simulink library "lib_transmission2"  (Simulink 4.1.1)
values from neighbouring files (symbols this model uses):
  logFlag = 1    [advSACompMaskInit.m]    (also in advSACompMaskInitR13.m)
undefined symbols (not defined in the file or in its folder): cyc_mph, fc_map_spd, fc_max_trq, fc_spd_scale, fc_trq_scale, fd_inertia, fd_loss, fd_ratio, gb_dnshift_load, gb_dnshift_spd, gb_gear_number_lookup, gb_gears_num, gb_inertia, gb_loss_const, gb_loss_input_spd_coeff, gb_loss_input_trq_coeff, gb_loss_output_spd_coeff, gb_loss_output_trq_coeff, gb_map_spd_out, gb_map_trq_in, gb_map_trq_out, gb_num_init, gb_ratio, gb_shift_delay, gb_spd_scale, gb_trq_scale, gb_upshift_load, gb_upshift_spd, htc_inertia, htc_k_adv, htc_k_adv_coast, htc_lockup, htc_lockup_load, htc_lockup_spd, htc_lu_gear_range, htc_max_coast_tr, htc_min_coast_tr, htc_pump_loss_spd, htc_pump_loss_trq_lockup, htc_pump_loss_trq_unlock, htc_sr, htc_sr_coast, htc_tr, htc_tr_coast, htc_unlock_spd, mc_map_spd, mc_max_trq, mc_overtrq_factor, mc_spd_scale, mc_trq_scale, tc_loss, tc_mc_to_fc_ratio, tx_eff_map, tx_map_spd, tx_map_trq, tx_pg_r, tx_pg_s, tx_speed_dep, vc_clutch_bool, vc_idle_spd ... (+2)
libraries: lib_controls x1, lib_etc x1, lib_controls2 x1, lib_transmission x1
(part 7 of 17)

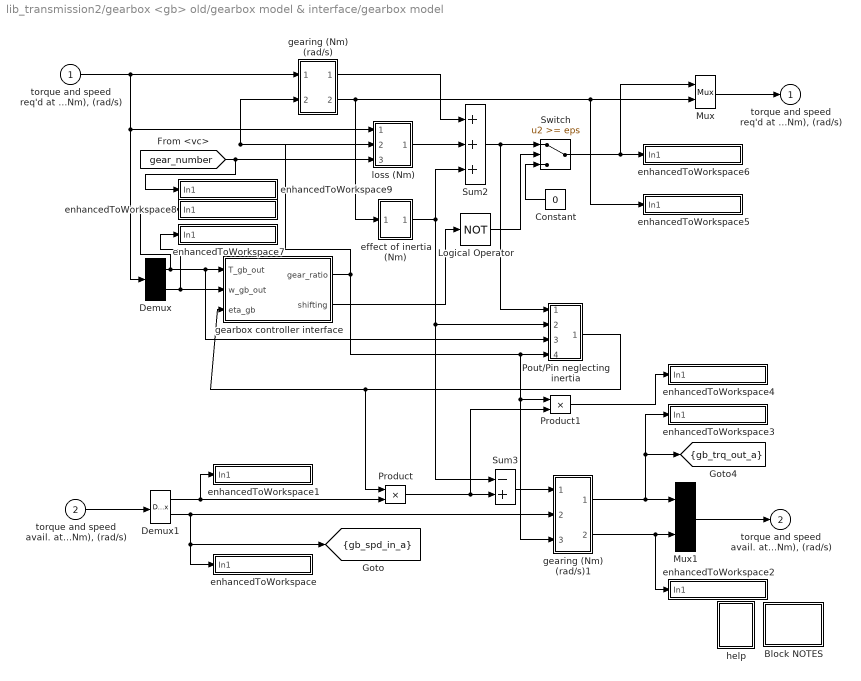
== system lib_transmission2/gearbox <gb> old/gearbox model & interface/gearbox model ==
  "torque and speed req'd at output side of gearbox (Nm), (rad/s)" : Inport  Port=1  LatchInput=off
  "torque and speed avail. at input side of gearbox (Nm), (rad/s)" : Inport  Port=2  LatchInput=off
  Block NOTES : Subsystem
      settings: RTWFcnNameOpts=Auto  RTWFileNameOpts=Auto
      mask Display: disp('Block\nNOTES')
  Constant : Constant  Orientation=left  Value=0
  Demux : Demux  Outputs=2  BusSelectionMode=off
  Demux1 : Demux  Outputs=2  BusSelectionMode=off
  Logical Operator : Logic  Operator=NOT  Inputs=1
  Mux : Mux  Inputs=2
      settings: DisplayOption=none
  Mux1 : Mux  Inputs=2
      settings: DisplayOption=none
  Pout/Pin neglecting inertia : Subsystem
      settings: RTWFcnNameOpts=Auto  RTWFileNameOpts=Auto
  Product : Product  Inputs=2  Multiplication=Element-wise(.*)  SaturateOnIntegerOverflow=on
  Product1 : Product  Inputs=2  Multiplication=Element-wise(.*)  SaturateOnIntegerOverflow=on
  Sum2 : Sum  Inputs=+++  SaturateOnIntegerOverflow=on
  Sum3 : Sum  Inputs=-+  SaturateOnIntegerOverflow=on
  Switch : Switch  Threshold=eps
  effect of inertia (Nm) : Subsystem
      settings: RTWFcnNameOpts=Auto  RTWFileNameOpts=Auto
  enhancedToWorkspace : Subsystem  mask(enhancedToWorkspace){generalName=generalName, specificName=spd_in_a, logFlag=logFlag}
      mask prompts: generalName "General Name [char-evaluated]"; specificName "Specific Name [char-literal]"; logFlag "Enable flag (1=on,0=off)"
      mask help: A wrapper for the Simulink "To Workspace" block that allows you to evaluate the name of the variable to log to workspace. This is useful to avoid the double logging errors that occur when you pull in two library models that attempt to log to the same variable.
      mask init:
      | enhancedToWsMaker
      settings: CopyFcn=breakLinkCopyFcn  ParentCloseFcn=breakLinkParCloseFcn  RTWFcnNameOpts=Auto  RTWFileNameOpts=Auto
      mask Help:
      | <h2>Enhanced To Workspace Block</h2>
      | <h3>Parameters</h3>
      | <UL>
      | <li><b>General Name:</b> This is the more general name of the variable. Variables are saved to the workspace as <i>generalName_specificName</i>. Note that this is an evaluated variable. If you would like to type in the value directly, it must be surrounded with single quotes. Otherwise you can input the name of a variable containing a char string.</li>
      | <li><b>Specific Name:</b> This is the specific name of the variable. Note that this is input as a char literal (i.e., you don't need quotes).</li>
      | <li><b>Enable Flag:</b> This flag should have the value of 0 or 1. If 0, the variable will not be logged to the workspace. If 1, the variable will be logged. This is done so that variable logging can be turned off to improve speed.</li>
      | </ul>
      | <h3>Overview</h3>
      | <p>The enhanced to workspace block was put together to allow one to dynamically resolve variable names at run time in simulink. This is most powerful when used in conjunction with a masked subsystem to allow multiple instances of that masked subsytem to be used in the same model. The strategy is to set the generalName in the block mask which will allow the block to change the general name for all variable logging on the fly.
      | <h3>Helper Files</h3>
      | <p>Three m-files are required by the enhancedToWorkspace block. These files are located in the &lt; ADVISOR root &gt;/GUI directory :
      | <ul>
      | <li><i>enhancedToWsMaker.m</i> This file runs the mask initialization for the block</li>
      | <li><i>breakLinkCopyFcn.m</i> This file is used by the block callback when the simulink block is copied. It is necessary to break the link to the enhancedToWorkspace similar to the To Workspace block in order for it to be able to configure itself. (Try copying simulink's To Workspace block--it is impossible to make a link)</li>
      | <li><i>breakLinkParCloseFcn.m</i> This file is similar to the breakLinkCopyFcn and is used when a parent system is closed</li>
      | </ul>
      | <hr>
      | 
      | <p>Created 2003-Jan-21, Michael Patrick O'Keefe, NREL</p>
      mask Display: disp([generalName,'_',specificName])
  enhancedToWorkspace1 : Subsystem  mask(enhancedToWorkspace){generalName=generalName, specificName=trq_in_a, logFlag=logFlag}
      mask prompts: generalName "General Name [char-evaluated]"; specificName "Specific Name [char-literal]"; logFlag "Enable flag (1=on,0=off)"
      mask help: A wrapper for the Simulink "To Workspace" block that allows you to evaluate the name of the variable to log to workspace. This is useful to avoid the double logging errors that occur when you pull in two library models that attempt to log to the same variable.
      mask init:
      | enhancedToWsMaker
      settings: CopyFcn=breakLinkCopyFcn  ParentCloseFcn=breakLinkParCloseFcn  RTWFcnNameOpts=Auto  RTWFileNameOpts=Auto
      mask Help:
      | <h2>Enhanced To Workspace Block</h2>
      | <h3>Parameters</h3>
      | <UL>
      | <li><b>General Name:</b> This is the more general name of the variable. Variables are saved to the workspace as <i>generalName_specificName</i>. Note that this is an evaluated variable. If you would like to type in the value directly, it must be surrounded with single quotes. Otherwise you can input the name of a variable containing a char string.</li>
      | <li><b>Specific Name:</b> This is the specific name of the variable. Note that this is input as a char literal (i.e., you don't need quotes).</li>
      | <li><b>Enable Flag:</b> This flag should have the value of 0 or 1. If 0, the variable will not be logged to the workspace. If 1, the variable will be logged. This is done so that variable logging can be turned off to improve speed.</li>
      | </ul>
      | <h3>Overview</h3>
      | <p>The enhanced to workspace block was put together to allow one to dynamically resolve variable names at run time in simulink. This is most powerful when used in conjunction with a masked subsystem to allow multiple instances of that masked subsytem to be used in the same model. The strategy is to set the generalName in the block mask which will allow the block to change the general name for all variable logging on the fly.
      | <h3>Helper Files</h3>
      | <p>Three m-files are required by the enhancedToWorkspace block. These files are located in the &lt; ADVISOR root &gt;/GUI directory :
      | <ul>
      | <li><i>enhancedToWsMaker.m</i> This file runs the mask initialization for the block</li>
      | <li><i>breakLinkCopyFcn.m</i> This file is used by the block callback when the simulink block is copied. It is necessary to break the link to the enhancedToWorkspace similar to the To Workspace block in order for it to be able to configure itself. (Try copying simulink's To Workspace block--it is impossible to make a link)</li>
      | <li><i>breakLinkParCloseFcn.m</i> This file is similar to the breakLinkCopyFcn and is used when a parent system is closed</li>
      | </ul>
      | <hr>
      | 
      | <p>Created 2003-Jan-21, Michael Patrick O'Keefe, NREL</p>
      mask Display: disp([generalName,'_',specificName])
  enhancedToWorkspace2 : Subsystem  mask(enhancedToWorkspace){generalName=generalName, specificName=spd_out_a, logFlag=logFlag}
      mask prompts: generalName "General Name [char-evaluated]"; specificName "Specific Name [char-literal]"; logFlag "Enable flag (1=on,0=off)"
      mask help: A wrapper for the Simulink "To Workspace" block that allows you to evaluate the name of the variable to log to workspace. This is useful to avoid the double logging errors that occur when you pull in two library models that attempt to log to the same variable.
      mask init:
      | enhancedToWsMaker
      settings: CopyFcn=breakLinkCopyFcn  ParentCloseFcn=breakLinkParCloseFcn  RTWFcnNameOpts=Auto  RTWFileNameOpts=Auto
      mask Help:
      | <h2>Enhanced To Workspace Block</h2>
      | <h3>Parameters</h3>
      | <UL>
      | <li><b>General Name:</b> This is the more general name of the variable. Variables are saved to the workspace as <i>generalName_specificName</i>. Note that this is an evaluated variable. If you would like to type in the value directly, it must be surrounded with single quotes. Otherwise you can input the name of a variable containing a char string.</li>
      | <li><b>Specific Name:</b> This is the specific name of the variable. Note that this is input as a char literal (i.e., you don't need quotes).</li>
      | <li><b>Enable Flag:</b> This flag should have the value of 0 or 1. If 0, the variable will not be logged to the workspace. If 1, the variable will be logged. This is done so that variable logging can be turned off to improve speed.</li>
      | </ul>
      | <h3>Overview</h3>
      | <p>The enhanced to workspace block was put together to allow one to dynamically resolve variable names at run time in simulink. This is most powerful when used in conjunction with a masked subsystem to allow multiple instances of that masked subsytem to be used in the same model. The strategy is to set the generalName in the block mask which will allow the block to change the general name for all variable logging on the fly.
      | <h3>Helper Files</h3>
      | <p>Three m-files are required by the enhancedToWorkspace block. These files are located in the &lt; ADVISOR root &gt;/GUI directory :
      | <ul>
      | <li><i>enhancedToWsMaker.m</i> This file runs the mask initialization for the block</li>
      | <li><i>breakLinkCopyFcn.m</i> This file is used by the block callback when the simulink block is copied. It is necessary to break the link to the enhancedToWorkspace similar to the To Workspace block in order for it to be able to configure itself. (Try copying simulink's To Workspace block--it is impossible to make a link)</li>
      | <li><i>breakLinkParCloseFcn.m</i> This file is similar to the breakLinkCopyFcn and is used when a parent system is closed</li>
      | </ul>
      | <hr>
      | 
      | <p>Created 2003-Jan-21, Michael Patrick O'Keefe, NREL</p>
      mask Display: disp([generalName,'_',specificName])
  enhancedToWorkspace3 : Subsystem  mask(enhancedToWorkspace){generalName=generalName, specificName=trq_out_a, logFlag=logFlag}
      mask prompts: generalName "General Name [char-evaluated]"; specificName "Specific Name [char-literal]"; logFlag "Enable flag (1=on,0=off)"
      mask help: A wrapper for the Simulink "To Workspace" block that allows you to evaluate the name of the variable to log to workspace. This is useful to avoid the double logging errors that occur when you pull in two library models that attempt to log to the same variable.
      mask init:
      | enhancedToWsMaker
      settings: CopyFcn=breakLinkCopyFcn  ParentCloseFcn=breakLinkParCloseFcn  RTWFcnNameOpts=Auto  RTWFileNameOpts=Auto
      mask Help:
      | <h2>Enhanced To Workspace Block</h2>
      | <h3>Parameters</h3>
      | <UL>
      | <li><b>General Name:</b> This is the more general name of the variable. Variables are saved to the workspace as <i>generalName_specificName</i>. Note that this is an evaluated variable. If you would like to type in the value directly, it must be surrounded with single quotes. Otherwise you can input the name of a variable containing a char string.</li>
      | <li><b>Specific Name:</b> This is the specific name of the variable. Note that this is input as a char literal (i.e., you don't need quotes).</li>
      | <li><b>Enable Flag:</b> This flag should have the value of 0 or 1. If 0, the variable will not be logged to the workspace. If 1, the variable will be logged. This is done so that variable logging can be turned off to improve speed.</li>
      | </ul>
      | <h3>Overview</h3>
      | <p>The enhanced to workspace block was put together to allow one to dynamically resolve variable names at run time in simulink. This is most powerful when used in conjunction with a masked subsystem to allow multiple instances of that masked subsytem to be used in the same model. The strategy is to set the generalName in the block mask which will allow the block to change the general name for all variable logging on the fly.
      | <h3>Helper Files</h3>
      | <p>Three m-files are required by the enhancedToWorkspace block. These files are located in the &lt; ADVISOR root &gt;/GUI directory :
      | <ul>
      | <li><i>enhancedToWsMaker.m</i> This file runs the mask initialization for the block</li>
      | <li><i>breakLinkCopyFcn.m</i> This file is used by the block callback when the simulink block is copied. It is necessary to break the link to the enhancedToWorkspace similar to the To Workspace block in order for it to be able to configure itself. (Try copying simulink's To Workspace block--it is impossible to make a link)</li>
      | <li><i>breakLinkParCloseFcn.m</i> This file is similar to the breakLinkCopyFcn and is used when a parent system is closed</li>
      | </ul>
      | <hr>
      | 
      | <p>Created 2003-Jan-21, Michael Patrick O'Keefe, NREL</p>
      mask Display: disp([generalName,'_',specificName])
  enhancedToWorkspace4 : Subsystem  mask(enhancedToWorkspace){generalName=generalName, specificName=ni_trq_out_a, logFlag=logFlag}
      mask prompts: generalName "General Name [char-evaluated]"; specificName "Specific Name [char-literal]"; logFlag "Enable flag (1=on,0=off)"
      mask help: A wrapper for the Simulink "To Workspace" block that allows you to evaluate the name of the variable to log to workspace. This is useful to avoid the double logging errors that occur when you pull in two library models that attempt to log to the same variable.
      mask init:
      | enhancedToWsMaker
      settings: CopyFcn=breakLinkCopyFcn  ParentCloseFcn=breakLinkParCloseFcn  RTWFcnNameOpts=Auto  RTWFileNameOpts=Auto
      mask Help:
      | <h2>Enhanced To Workspace Block</h2>
      | <h3>Parameters</h3>
      | <UL>
      | <li><b>General Name:</b> This is the more general name of the variable. Variables are saved to the workspace as <i>generalName_specificName</i>. Note that this is an evaluated variable. If you would like to type in the value directly, it must be surrounded with single quotes. Otherwise you can input the name of a variable containing a char string.</li>
      | <li><b>Specific Name:</b> This is the specific name of the variable. Note that this is input as a char literal (i.e., you don't need quotes).</li>
      | <li><b>Enable Flag:</b> This flag should have the value of 0 or 1. If 0, the variable will not be logged to the workspace. If 1, the variable will be logged. This is done so that variable logging can be turned off to improve speed.</li>
      | </ul>
      | <h3>Overview</h3>
      | <p>The enhanced to workspace block was put together to allow one to dynamically resolve variable names at run time in simulink. This is most powerful when used in conjunction with a masked subsystem to allow multiple instances of that masked subsytem to be used in the same model. The strategy is to set the generalName in the block mask which will allow the block to change the general name for all variable logging on the fly.
      | <h3>Helper Files</h3>
      | <p>Three m-files are required by the enhancedToWorkspace block. These files are located in the &lt; ADVISOR root &gt;/GUI directory :
      | <ul>
      | <li><i>enhancedToWsMaker.m</i> This file runs the mask initialization for the block</li>
      | <li><i>breakLinkCopyFcn.m</i> This file is used by the block callback when the simulink block is copied. It is necessary to break the link to the enhancedToWorkspace similar to the To Workspace block in order for it to be able to configure itself. (Try copying simulink's To Workspace block--it is impossible to make a link)</li>
      | <li><i>breakLinkParCloseFcn.m</i> This file is similar to the breakLinkCopyFcn and is used when a parent system is closed</li>
      | </ul>
      | <hr>
      | 
      | <p>Created 2003-Jan-21, Michael Patrick O'Keefe, NREL</p>
      mask Display: disp([generalName,'_',specificName])
  enhancedToWorkspace5 : Subsystem  mask(enhancedToWorkspace){generalName=generalName, specificName=spd_in_r, logFlag=logFlag}
      mask prompts: generalName "General Name [char-evaluated]"; specificName "Specific Name [char-literal]"; logFlag "Enable flag (1=on,0=off)"
      mask help: A wrapper for the Simulink "To Workspace" block that allows you to evaluate the name of the variable to log to workspace. This is useful to avoid the double logging errors that occur when you pull in two library models that attempt to log to the same variable.
      mask init:
      | enhancedToWsMaker
      settings: CopyFcn=breakLinkCopyFcn  ParentCloseFcn=breakLinkParCloseFcn  RTWFcnNameOpts=Auto  RTWFileNameOpts=Auto
      mask Help:
      | <h2>Enhanced To Workspace Block</h2>
      | <h3>Parameters</h3>
      | <UL>
      | <li><b>General Name:</b> This is the more general name of the variable. Variables are saved to the workspace as <i>generalName_specificName</i>. Note that this is an evaluated variable. If you would like to type in the value directly, it must be surrounded with single quotes. Otherwise you can input the name of a variable containing a char string.</li>
      | <li><b>Specific Name:</b> This is the specific name of the variable. Note that this is input as a char literal (i.e., you don't need quotes).</li>
      | <li><b>Enable Flag:</b> This flag should have the value of 0 or 1. If 0, the variable will not be logged to the workspace. If 1, the variable will be logged. This is done so that variable logging can be turned off to improve speed.</li>
      | </ul>
      | <h3>Overview</h3>
      | <p>The enhanced to workspace block was put together to allow one to dynamically resolve variable names at run time in simulink. This is most powerful when used in conjunction with a masked subsystem to allow multiple instances of that masked subsytem to be used in the same model. The strategy is to set the generalName in the block mask which will allow the block to change the general name for all variable logging on the fly.
      | <h3>Helper Files</h3>
      | <p>Three m-files are required by the enhancedToWorkspace block. These files are located in the &lt; ADVISOR root &gt;/GUI directory :
      | <ul>
      | <li><i>enhancedToWsMaker.m</i> This file runs the mask initialization for the block</li>
      | <li><i>breakLinkCopyFcn.m</i> This file is used by the block callback when the simulink block is copied. It is necessary to break the link to the enhancedToWorkspace similar to the To Workspace block in order for it to be able to configure itself. (Try copying simulink's To Workspace block--it is impossible to make a link)</li>
      | <li><i>breakLinkParCloseFcn.m</i> This file is similar to the breakLinkCopyFcn and is used when a parent system is closed</li>
      | </ul>
      | <hr>
      | 
      | <p>Created 2003-Jan-21, Michael Patrick O'Keefe, NREL</p>
      mask Display: disp([generalName,'_',specificName])
  enhancedToWorkspace6 : Subsystem  mask(enhancedToWorkspace){generalName=generalName, specificName=trq_in_r, logFlag=logFlag}
      mask prompts: generalName "General Name [char-evaluated]"; specificName "Specific Name [char-literal]"; logFlag "Enable flag (1=on,0=off)"
      mask help: A wrapper for the Simulink "To Workspace" block that allows you to evaluate the name of the variable to log to workspace. This is useful to avoid the double logging errors that occur when you pull in two library models that attempt to log to the same variable.
      mask init:
      | enhancedToWsMaker
      settings: CopyFcn=breakLinkCopyFcn  ParentCloseFcn=breakLinkParCloseFcn  RTWFcnNameOpts=Auto  RTWFileNameOpts=Auto
      mask Help:
      | <h2>Enhanced To Workspace Block</h2>
      | <h3>Parameters</h3>
      | <UL>
      | <li><b>General Name:</b> This is the more general name of the variable. Variables are saved to the workspace as <i>generalName_specificName</i>. Note that this is an evaluated variable. If you would like to type in the value directly, it must be surrounded with single quotes. Otherwise you can input the name of a variable containing a char string.</li>
      | <li><b>Specific Name:</b> This is the specific name of the variable. Note that this is input as a char literal (i.e., you don't need quotes).</li>
      | <li><b>Enable Flag:</b> This flag should have the value of 0 or 1. If 0, the variable will not be logged to the workspace. If 1, the variable will be logged. This is done so that variable logging can be turned off to improve speed.</li>
      | </ul>
      | <h3>Overview</h3>
      | <p>The enhanced to workspace block was put together to allow one to dynamically resolve variable names at run time in simulink. This is most powerful when used in conjunction with a masked subsystem to allow multiple instances of that masked subsytem to be used in the same model. The strategy is to set the generalName in the block mask which will allow the block to change the general name for all variable logging on the fly.
      | <h3>Helper Files</h3>
      | <p>Three m-files are required by the enhancedToWorkspace block. These files are located in the &lt; ADVISOR root &gt;/GUI directory :
      | <ul>
      | <li><i>enhancedToWsMaker.m</i> This file runs the mask initialization for the block</li>
      | <li><i>breakLinkCopyFcn.m</i> This file is used by the block callback when the simulink block is copied. It is necessary to break the link to the enhancedToWorkspace similar to the To Workspace block in order for it to be able to configure itself. (Try copying simulink's To Workspace block--it is impossible to make a link)</li>
      | <li><i>breakLinkParCloseFcn.m</i> This file is similar to the breakLinkCopyFcn and is used when a parent system is closed</li>
      | </ul>
      | <hr>
      | 
      | <p>Created 2003-Jan-21, Michael Patrick O'Keefe, NREL</p>
      mask Display: disp([generalName,'_',specificName])
  enhancedToWorkspace7 : Subsystem  mask(enhancedToWorkspace){generalName=generalName, specificName=spd_out_r, logFlag=logFlag}
      mask prompts: generalName "General Name [char-evaluated]"; specificName "Specific Name [char-literal]"; logFlag "Enable flag (1=on,0=off)"
      mask help: A wrapper for the Simulink "To Workspace" block that allows you to evaluate the name of the variable to log to workspace. This is useful to avoid the double logging errors that occur when you pull in two library models that attempt to log to the same variable.
      mask init:
      | enhancedToWsMaker
      settings: CopyFcn=breakLinkCopyFcn  ParentCloseFcn=breakLinkParCloseFcn  RTWFcnNameOpts=Auto  RTWFileNameOpts=Auto
      mask Help:
      | <h2>Enhanced To Workspace Block</h2>
      | <h3>Parameters</h3>
      | <UL>
      | <li><b>General Name:</b> This is the more general name of the variable. Variables are saved to the workspace as <i>generalName_specificName</i>. Note that this is an evaluated variable. If you would like to type in the value directly, it must be surrounded with single quotes. Otherwise you can input the name of a variable containing a char string.</li>
      | <li><b>Specific Name:</b> This is the specific name of the variable. Note that this is input as a char literal (i.e., you don't need quotes).</li>
      | <li><b>Enable Flag:</b> This flag should have the value of 0 or 1. If 0, the variable will not be logged to the workspace. If 1, the variable will be logged. This is done so that variable logging can be turned off to improve speed.</li>
      | </ul>
      | <h3>Overview</h3>
      | <p>The enhanced to workspace block was put together to allow one to dynamically resolve variable names at run time in simulink. This is most powerful when used in conjunction with a masked subsystem to allow multiple instances of that masked subsytem to be used in the same model. The strategy is to set the generalName in the block mask which will allow the block to change the general name for all variable logging on the fly.
      | <h3>Helper Files</h3>
      | <p>Three m-files are required by the enhancedToWorkspace block. These files are located in the &lt; ADVISOR root &gt;/GUI directory :
      | <ul>
      | <li><i>enhancedToWsMaker.m</i> This file runs the mask initialization for the block</li>
      | <li><i>breakLinkCopyFcn.m</i> This file is used by the block callback when the simulink block is copied. It is necessary to break the link to the enhancedToWorkspace similar to the To Workspace block in order for it to be able to configure itself. (Try copying simulink's To Workspace block--it is impossible to make a link)</li>
      | <li><i>breakLinkParCloseFcn.m</i> This file is similar to the breakLinkCopyFcn and is used when a parent system is closed</li>
      | </ul>
      | <hr>
      | 
      | <p>Created 2003-Jan-21, Michael Patrick O'Keefe, NREL</p>
      mask Display: disp([generalName,'_',specificName])
  enhancedToWorkspace8 : Subsystem  mask(enhancedToWorkspace){generalName=generalName, specificName=trq_out_r, logFlag=logFlag}
      mask prompts: generalName "General Name [char-evaluated]"; specificName "Specific Name [char-literal]"; logFlag "Enable flag (1=on,0=off)"
      mask help: A wrapper for the Simulink "To Workspace" block that allows you to evaluate the name of the variable to log to workspace. This is useful to avoid the double logging errors that occur when you pull in two library models that attempt to log to the same variable.
      mask init:
      | enhancedToWsMaker
      settings: CopyFcn=breakLinkCopyFcn  ParentCloseFcn=breakLinkParCloseFcn  RTWFcnNameOpts=Auto  RTWFileNameOpts=Auto
      mask Help:
      | <h2>Enhanced To Workspace Block</h2>
      | <h3>Parameters</h3>
      | <UL>
      | <li><b>General Name:</b> This is the more general name of the variable. Variables are saved to the workspace as <i>generalName_specificName</i>. Note that this is an evaluated variable. If you would like to type in the value directly, it must be surrounded with single quotes. Otherwise you can input the name of a variable containing a char string.</li>
      | <li><b>Specific Name:</b> This is the specific name of the variable. Note that this is input as a char literal (i.e., you don't need quotes).</li>
      | <li><b>Enable Flag:</b> This flag should have the value of 0 or 1. If 0, the variable will not be logged to the workspace. If 1, the variable will be logged. This is done so that variable logging can be turned off to improve speed.</li>
      | </ul>
      | <h3>Overview</h3>
      | <p>The enhanced to workspace block was put together to allow one to dynamically resolve variable names at run time in simulink. This is most powerful when used in conjunction with a masked subsystem to allow multiple instances of that masked subsytem to be used in the same model. The strategy is to set the generalName in the block mask which will allow the block to change the general name for all variable logging on the fly.
      | <h3>Helper Files</h3>
      | <p>Three m-files are required by the enhancedToWorkspace block. These files are located in the &lt; ADVISOR root &gt;/GUI directory :
      | <ul>
      | <li><i>enhancedToWsMaker.m</i> This file runs the mask initialization for the block</li>
      | <li><i>breakLinkCopyFcn.m</i> This file is used by the block callback when the simulink block is copied. It is necessary to break the link to the enhancedToWorkspace similar to the To Workspace block in order for it to be able to configure itself. (Try copying simulink's To Workspace block--it is impossible to make a link)</li>
      | <li><i>breakLinkParCloseFcn.m</i> This file is similar to the breakLinkCopyFcn and is used when a parent system is closed</li>
      | </ul>
      | <hr>
      | 
      | <p>Created 2003-Jan-21, Michael Patrick O'Keefe, NREL</p>
      mask Display: disp([generalName,'_',specificName])
  enhancedToWorkspace9 : Subsystem  mask(enhancedToWorkspace){generalName=generalName, specificName=gear_number, logFlag=logFlag}
      mask prompts: generalName "General Name [char-evaluated]"; specificName "Specific Name [char-literal]"; logFlag "Enable flag (1=on,0=off)"
      mask help: A wrapper for the Simulink "To Workspace" block that allows you to evaluate the name of the variable to log to workspace. This is useful to avoid the double logging errors that occur when you pull in two library models that attempt to log to the same variable.
      mask init:
      | enhancedToWsMaker
      settings: CopyFcn=breakLinkCopyFcn  ParentCloseFcn=breakLinkParCloseFcn  RTWFcnNameOpts=Auto  RTWFileNameOpts=Auto
      mask Help:
      | <h2>Enhanced To Workspace Block</h2>
      | <h3>Parameters</h3>
      | <UL>
      | <li><b>General Name:</b> This is the more general name of the variable. Variables are saved to the workspace as <i>generalName_specificName</i>. Note that this is an evaluated variable. If you would like to type in the value directly, it must be surrounded with single quotes. Otherwise you can input the name of a variable containing a char string.</li>
      | <li><b>Specific Name:</b> This is the specific name of the variable. Note that this is input as a char literal (i.e., you don't need quotes).</li>
      | <li><b>Enable Flag:</b> This flag should have the value of 0 or 1. If 0, the variable will not be logged to the workspace. If 1, the variable will be logged. This is done so that variable logging can be turned off to improve speed.</li>
      | </ul>
      | <h3>Overview</h3>
      | <p>The enhanced to workspace block was put together to allow one to dynamically resolve variable names at run time in simulink. This is most powerful when used in conjunction with a masked subsystem to allow multiple instances of that masked subsytem to be used in the same model. The strategy is to set the generalName in the block mask which will allow the block to change the general name for all variable logging on the fly.
      | <h3>Helper Files</h3>
      | <p>Three m-files are required by the enhancedToWorkspace block. These files are located in the &lt; ADVISOR root &gt;/GUI directory :
      | <ul>
      | <li><i>enhancedToWsMaker.m</i> This file runs the mask initialization for the block</li>
      | <li><i>breakLinkCopyFcn.m</i> This file is used by the block callback when the simulink block is copied. It is necessary to break the link to the enhancedToWorkspace similar to the To Workspace block in order for it to be able to configure itself. (Try copying simulink's To Workspace block--it is impossible to make a link)</li>
      | <li><i>breakLinkParCloseFcn.m</i> This file is similar to the breakLinkCopyFcn and is used when a parent system is closed</li>
      | </ul>
      | <hr>
      | 
      | <p>Created 2003-Jan-21, Michael Patrick O'Keefe, NREL</p>
      mask Display: disp([generalName,'_',specificName])
  gearbox controller interface : Subsystem
      settings: RTWFcnNameOpts=Auto  RTWFileNameOpts=Auto
  gearing (Nm) (rad/s) : Subsystem
      settings: RTWFcnNameOpts=Auto  RTWFileNameOpts=Auto
  gearing (Nm) (rad/s)1 : Subsystem
      settings: RTWFcnNameOpts=Auto  RTWFileNameOpts=Auto
  help : Subsystem
      settings: OpenFcn=web(['file:\\\' which('gearbox.htm')]);  RTWFcnNameOpts=Auto  RTWFileNameOpts=Auto
      mask Display: image(imread('doc_man.jpg'))
  loss (Nm) : Subsystem  mask{tx_eff_map=tx_eff_map, tx_map_trq=tx_map_trq, tx_map_spd=tx_map_spd, gb_spd_scale=gb_spd_scale, gb_trq_scale=gb_trq_scale}
      mask prompts: tx_eff_map "table of efficiency values (spd rad/s, trq Nm)"; tx_map_trq "vector of output torque values for lookup table (Nm)"; tx_map_spd "vector of output speeds for lookup table (rad/s)"; gb_spd_scale "Speed scale for the transmission gear box"; gb_trq_scale "Torque scale for the transmission gear box"
      settings: RTWFcnNameOpts=Auto  RTWFileNameOpts=Auto
  "torque and speed req'd at input side of gearbox (Nm), (rad/s)" : Outport  Port=1  InitialOutput=0
  "torque and speed avail. at output side of gearbox (Nm), (rad/s)" : Outport  Port=2  InitialOutput=0
  tag scope: gb_spd_in_a=scoped, gb_trq_out_a=scoped
  wires:
  gearbox controller interface/1(gear_ratio) -> Product1/1, gearing (Nm) (rad/s)1/3(gear ratio), Pout/Pin neglecting inertia/4(gear ratio), gearing (Nm) (rad/s)/2(gear ratio), loss (Nm)/2(gear ratio)
  loss (Nm)/1(loss torque at input shaft (Nm)) -> Sum2/2
  Constant/1 -> Switch/3
  Switch/1 -> Mux/1, enhancedToWorkspace6/1(In1)
  Logical Operator/1 -> Switch/2
  gearbox controller interface/2(shifting) -> Logical Operator/1
  Sum2/1 -> Switch/1, Pout/Pin neglecting inertia/1(Tin)
  Demux1/2 -> [gb_spd_in_a], enhancedToWorkspace/1(In1), gearing (Nm) (rad/s)1/2(input shaft speed (rad/s))
  Demux1/1 -> Product/2, enhancedToWorkspace1/1(In1)
  gearing (Nm) (rad/s)1/1(output shaft torque (Nm)) -> Mux1/1, enhancedToWorkspace3/1(In1), [gb_trq_out_a]
  gearing (Nm) (rad/s)1/2(output shaft speed (rad/s)) -> Mux1/2, enhancedToWorkspace2/1(In1)
  Demux/1 -> gearbox controller interface/1(T_gb_out), Pout/Pin neglecting inertia/3(Tout), enhancedToWorkspace8/1(In1)
  Demux/2 -> gearbox controller interface/2(w_gb_out), enhancedToWorkspace7/1(In1)
  "torque and speed req'd at output side of gearbox (Nm), (rad/s)"/1 -> gearing (Nm) (rad/s)/1("output shaft torque and speed  (Nm), (rad/s)"), Demux/1, loss (Nm)/1("output torque and speed (Nm), (rad/s)")
  effect of inertia (Nm)/1(drag torque (Nm)) -> Sum3/1, Pout/Pin neglecting inertia/2(Tinertia), Sum2/3
  gearing (Nm) (rad/s)/2(input shaft speed (rad/s)) -> Mux/2, enhancedToWorkspace5/1(In1), effect of inertia (Nm)/1(gb input speed (rad/s))
  gearing (Nm) (rad/s)/1(input shaft torque (Nm)) -> Sum2/1
  Mux/1 -> "torque and speed req'd at input side of gearbox (Nm), (rad/s)"/1
  Pout/Pin neglecting inertia/1(Pout/Pin) -> Product/1, gearbox controller interface/3(eta_gb)
  "torque and speed avail. at input side of gearbox (Nm), (rad/s)"/1 -> Demux1/1
  Sum3/1 -> gearing (Nm) (rad/s)1/1(input shaft torque (Nm))
  Mux1/1 -> "torque and speed avail. at output side of gearbox (Nm), (rad/s)"/1
  Product/1 -> Sum3/2, Product1/2
  Product1/1 -> enhancedToWorkspace4/1(In1)
  [gear_number] -> enhancedToWorkspace9/1(In1), loss (Nm)/3(gear_number)

== system lib_transmission2/gearbox <gb> old/gearbox model & interface/signal annotator ==
  In1 : Inport  Port=1  LatchInput=off
  Demux : Demux  Outputs=2  BusSelectionMode=off
  Mux : Mux  Inputs=2
  Out1 : Outport  Port=1
  wires:
  In1/1 -> Demux/1
  Demux/1 -> Mux/1  "gb_trq_out_r"
  Demux/2 -> Mux/2  "gb_spd_out_r"
  Mux/1 -> Out1/1
